simulink model "simulacion_serial"  (R2016a)
settings: Solver=VariableStepAuto  SolverMode=SingleTasking  StartTime=0.0  StopTime=inf  RelTol=1e-3
libraries: mcbhostblockslib x3
settings Model: Creator=joseg  LastModifiedBy=joseg
settings DataIOCC: ReturnWorkspaceOutputs=on
settings DebuggingCC: SFUnexpectedBacktrackingDiag=error  SFNoUnconditionalDefaultTransitionDiag=error
settings SFSimCC: SimUseLocalCustomCode=on
settings RTWCC: RTWUseLocalCustomCode=on
settings GRTTargetCC: TargetLangStandard=C99 (ISO)
settings ConfigComp: CovMetricSettings=dwe  CovHtmlReporting=off  CovSaveCumulativeToWorkspaceVar=off  CovSaveSingleToWorkspaceVar=off  CovExternalEMLEnable=on

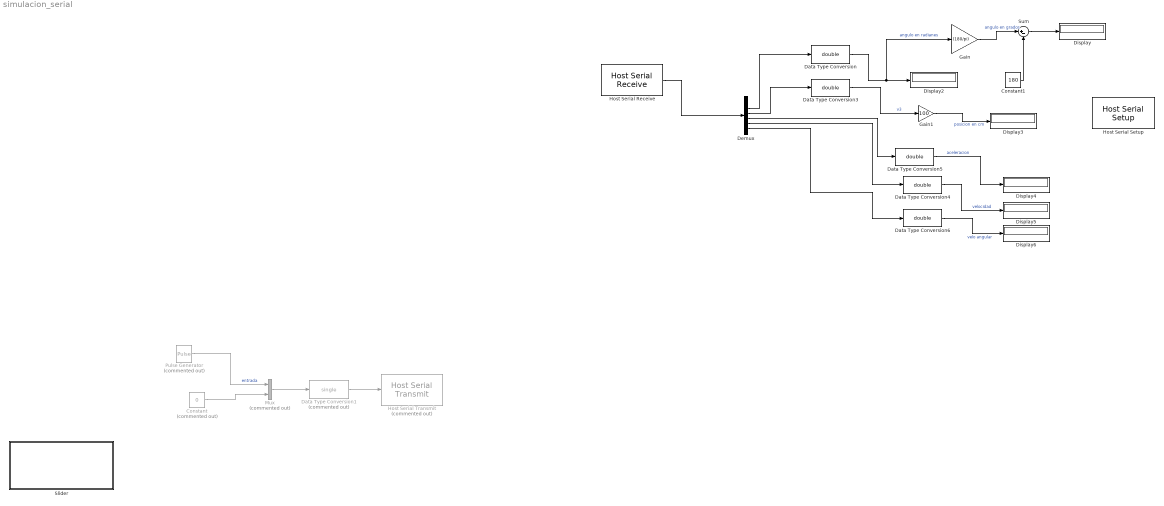
== system simulacion_serial ==
  Constant : Constant  Commented=on  Value=0
  Constant1 : Constant  Value=180
  Data Type Conversion{,3..6} (5 alike) : DataTypeConversion  OutDataTypeStr=double
  Data Type Conversion1 : DataTypeConversion  Commented=on  OutDataTypeStr=single
  Demux : Demux  Outputs=6
  Display{,2..6} (6 alike) : Display
  Gain : Gain  Gain=(180/pi)
  Gain1 : Gain  Gain=100
  Host Serial Receive : mcbhostblockslib/Host Serial Receive  serialCon=Serial 1  dataHead='V'  dataTail=[10]  dataType=single  dataDim=[6 1]  initValue=0  errOption=Output the last received value  errValue=0  sampleTime=0.01  outputStatus=off  blockingMode=on
  Host Serial Setup : mcbhostblockslib/Host Serial Setup  Priority=-99  comPortSer1='COM7'  baudRateA=115200  charLenA=8  stopBitA=1  parityA=none  timeoutA=10  ByteOrderA=LittleEndian  comPortSer2='Please_select_a_port'  baudRateB=115200  charLenB=8  stopBitB=1  parityB=none  timeoutB=1.0  ByteOrderB=LittleEndian  comPortSer3='Please_select_a_port'  baudRateC=115200  charLenC=8  stopBitC=1  parityC=none  timeoutC=1.0  ByteOrderC=LittleEndian  comPortSer4='Please_select_a_port'  baudRateD=115200  charLenD=8  stopBitD=1  parityD=none  timeoutD=1.0  ByteOrderD=LittleEndian
  Host Serial Transmit : mcbhostblockslib/Host Serial Transmit  Commented=on  serialCon=Serial 1  header=[]  tail=[]  enableBlockingMode=on
  Mux : Mux  Commented=on  Inputs=2
  Pulse Generator : DiscretePulseGenerator  Commented=on  PulseType=Time based  Period=1  PulseWidth=50
  Slider : Subsystem  DialogController=hmiCreateDDGDialog  IsWebBlock=on  mask(MWDashboardBlock){webBlockId=5397500b-7835-43e2-b6c4-527d1e3fb1e0, webBlockType=slider, ShowInLibBrowser=on, ShowInitialText=on, HMISrcModelName=simulacion_serial}
      mask prompts: webBlockId "WebBlock Id"; webBlockType "WebBlock Type"; HMISrcModelName "Source Model"
      mask help: Set value to tune parameters or variables.
      mask Help: helpview([docroot '/mapfiles/simulink.map'], 'hmi_slider')
      mask Display:
      | if strcmp(get_param(bdroot(gcb),'BlockDiagramType'),'library')
      |  image([(matlabroot) '/toolbox/simulink/hmi/icons/Slider.png'])
      | end
  Sum : Sum  Inputs=|+-
  wires:
  Host Serial Receive/1 -> Demux/1
  Data Type Conversion1/1 -> Host Serial Transmit/1
  Mux/1 -> Data Type Conversion1/1
  Pulse Generator/1 -> Mux/1  "entrada"
  Demux/2 -> Data Type Conversion/1
  Data Type Conversion/1 -> Gain/1, Display2/1  "angulo en radianes"
  Demux/3 -> Data Type Conversion3/1
  Data Type Conversion3/1 -> Gain1/1  "v3"
  Constant/1 -> Mux/2
  Demux/6 -> Data Type Conversion6/1
  Demux/5 -> Data Type Conversion4/1
  Data Type Conversion6/1 -> Display6/1  "velo angular"
  Data Type Conversion5/1 -> Display4/1  "aceleracion"
  Data Type Conversion4/1 -> Display5/1  "velocidad"
  Demux/4 -> Data Type Conversion5/1
  Gain1/1 -> Display3/1  "posicion en cm"
  Gain/1 -> Sum/1  "angulo en grados"
  Constant1/1 -> Sum/2
  Sum/1 -> Display/1

== system simulacion_serial/Slider ==
